simulink model "trajectory_gen2"  (R2020b)
settings: Solver=VariableStepAuto  StartTime=0.0  StopTime=400  RelTol=1e-3
libraries: robotcorelib x1
settings Model: Creator=shanerutherford  LastModifiedBy=shanerutherford

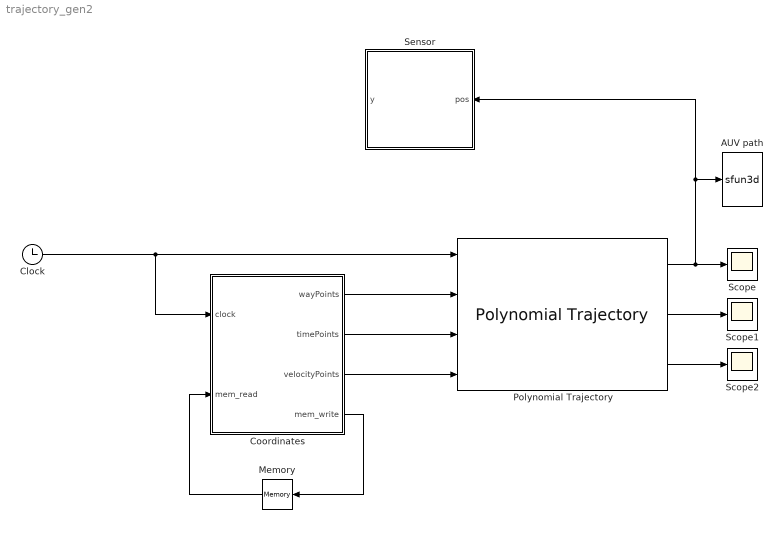
== system trajectory_gen2 ==
  AUV path : S-Function  LoadFcn=if exist('sfun3d','file'), sfun3d([],[],[],'LoadBlock'); end  FunctionName=sfun3d  Parameters=ax,T,np,cp,gd,ls,mk,mx,hd,tb  SFunctionDeploymentMode=off  EnableBusSupport=off  mask(3D Graph){np=1, ax=[-15 15 -15 15 -20 20], mx=1e4, T=1, cp=[0, 0 15], gd=on, hd=on, tb=on, ls=-, mk=none}
      mask prompts: np "Number of moving points (lines)"; ax "Range: [xmin xmax  ymin ymax zmin zmax]"; mx "Max number of points in each line"; T "Sampling Time"; cp "Camera position (use [0 0 1] for 2D XY view)"; gd "Grid (on|off)"; hd "HeadMarkers (on|off)"; tb "Toolbar (on|off)"; ls "LineStyle"; mk "LineMarker"
      mask help:
      | This block plots the position of several points in the XYZ space. The input contains the coordinates of all the points (x1,y1,z1,x2,y2,z2,...).
      | The number of moving points (lines), the XYZ ranges, sampling time, camera position, and grid (among other things) can be set as mask parameters.
      settings: CopyFcn=if exist('sfun3d','file'), sfun3d([],[],[],'CopyBlock'); end  DeleteFcn=if exist('sfun3d','file'), sfun3d([],[],[],'DeleteBlock'); end  NameChangeFcn=if exist('sfun3d','file'), sfun3d([],[],[],'NameChange'); end
      mask Help:
      | This block plots the position of several points in the XYZ space. The input contains the coordinates of all the points (x1,y1,z1,x2,y2,z2,...).
      | The number of moving points (lines), the XYZ ranges, sampling time, camera position, and grid (among other things) can be set as mask parameters.
      mask TypeOptions ls: - | -- | : | -. | none
      mask TypeOptions mk: none | . | + | o | * | x | square | diamond | v | ^ | > | < | pentagram | hexagram
      mask Display: plot([.05 .95 .95 .05 .05],[.45 .45 .95 .95 .45], 0.5+cos(0:0.1:2*pi)*0.3,0.7+sin(0:0.1:2*pi)*0.2)
  Clock : Clock
  Coordinates : MATLAB Function  TreatAsAtomicUnit=on
  Memory : Memory  InitialCondition=zeros(7, 7)
  Polynomial Trajectory : robotcorelib/Polynomial Trajectory  WaypointSource=External  Waypoints=[ 0, 2, 1, 5, 0; -1, 3, 1, 4, 4 ]  TimePoints=[ 0, 1, 2, 3, 4 ]  TimeInterval=[ 1, 4 ]  Method=Cubic Polynomial  ParameterSource=External  VelocityBoundaryCondition=zeros( 2, 5 )  AccelerationBoundaryCondition=zeros( 2, 5 )  SimulateUsing=Interpreted execution
  Scope : Scope
  Scope1 : Scope
  Scope2 : Scope
  Sensor : MATLAB Function  TreatAsAtomicUnit=on
  wires:
  Coordinates/4(mem_write) -> Memory/1
  Polynomial Trajectory/3 -> Scope2/1
  Polynomial Trajectory/2 -> Scope1/1
  Memory/1 -> Coordinates/2(mem_read)
  Clock/1 -> Coordinates/1(clock), Polynomial Trajectory/1
  Polynomial Trajectory/1 -> Scope/1, Sensor/1(pos), AUV path/1
  Coordinates/1(wayPoints) -> Polynomial Trajectory/2
  Coordinates/3(velocityPoints) -> Polynomial Trajectory/4
  Coordinates/2(timePoints) -> Polynomial Trajectory/3

== matlab function trajectory_gen2/Sensor ==
  data: pos input; y output
function y = fcn(pos)

y = u;

== matlab function trajectory_gen2/Coordinates ==
  data: wayPoints output; timePoints output; velocityPoints output; clock input; mem_read input; mem_write output
function [wayPoints, timePoints, velocityPoints, mem_write] = fcn(clock, mem_read)

    avg_speed = 0.8; % m/s
    
    % Should run one time to initalise waypoints
    if mem_read == 0
        wayPoints = [
            0, 10,   0, -10, 10,   0, -10;
            0, 10, -10,  10, 10, -10,  10;
            0,  0,   0,   0,  4,   4,   4; 
        ];
        timePoints = ones(1, 7);
        timePoints(1, 1) = 0;
        velocityPoints = zeros(3, 7);
    else
        wayPoints = mem_read(1:3, 1:7);
        timePoints = mem_read(4, 1:7);
        velocityPoints = mem_read(5:7, 1:7);
    end
    
    
    % generate a new random waypoint and rotate waypoints
    [~, n] = size(wayPoints);
    if clock > timePoints(1, 3)
        for i = 2:n
            wayPoints(1:3, i-1) = wayPoints(1:3, i);
            timePoints(1, i-1) = timePoints(1, i);
            velocityPoints(1:3, i-1) = velocityPoints(1:3, i);
        end
        wayPoints(1:3, n) = 20 * ([rand(1)-0.5; rand(1)-0.5; rand(1)-0.2]);
    end

    
    % Generate timepoints and velocity points
    for i = 2:n
        distance = norm(wayPoints(1:3, i) - wayPoints(1:3, i-1));
        timePoints(1, i) = timePoints(1, i-1) + distance/avg_speed;
    end
    
    for i = 2:n-1
        vector = wayPoints(1:3, i+1) - wayPoints(1:3, i-1);
        if abs(sum(vector)) < 0.1
            w = wayPoints(1:3, i) - wayPoints(1:3, i-1);
            vector = [-w(2); w(1); 0];
        end
        unit_d = vector / norm(vector);
        velocityPoints(1:3, i) = avg_speed*unit_d;
    end
    
    
    mem_write = [
        wayPoints; 
        timePoints;
        velocityPoints];
end
